simulink model "exercise75"  (Simulink 7.9)
settings: Solver=ode45  StartTime=0.0  StopTime=30  RelTol=1e-3
libraries: simulink x1
settings Model: Creator=esteur  LastModifiedBy=Chiscariu
settings OptimizationCC: InitFltsAndDblsToZero=on
settings DebuggingCC: FcnCallInpInsideContextMsg=Use local settings  StrictBusMsg=Warning
settings GRTTargetCC: CombineOutputUpdateFcns=off  GRTInterface=on

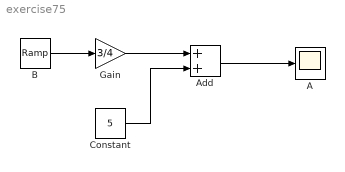
== system exercise75 ==
  A : Scope
      settings: TickLabels=on
  Add : Sum
  B : simulink/Sources/Ramp  slope=4  start=0  X0=0
  Constant : Constant  Value=5
  Gain : Gain  Gain=3/4
  wires:
  Gain/1 -> Add/1
  Constant/1 -> Add/2
  Add/1 -> A/1
  B/1 -> Gain/1
